simulink model "step6_3_setup_PID_test"  (R2021b)
settings: Solver=ode45  StartTime=0.0  StopTime=15  RelTol=1e-3  EnableMultiTasking=on
values from neighbouring files (symbols this model uses):
  adingain = [adin_gain 1 1 1 1 1]    [hwinit.m]    (also in hwinit_raw.m)
  adinoffs = [adin_offs 0 0 0 0 0]    [hwinit.m]    (also in hwinit_raw.m)
  daoutgain = 1*[-6]    [hwinit.m]    (also in hwinit_raw.m)
  daoutoffs = [0.00]    [hwinit.m]    (also in hwinit_raw.m)
  h = 0.001    [hwinit.m]    (also in hwinit_raw.m; init_fugi.m = fugiboard('Open', 'Pendulum1'); one_run.m = fugiboard('Open', 'pendulum1'); one_single_run.m = fugiboard('Open', 'pendulum1'))
  theta_1_0 = pi    (= 3.14159265359)    [hwinit.m]    (also in hwinit_raw.m; step4_0_linearize_operating_point.m; step5_observor_design.m = x_op(1); step6_1_controller_feedback.m = x_op(1))
  theta_2_0 = 0    [hwinit.m]    (also in hwinit_raw.m; step4_0_linearize_operating_point.m; step5_observor_design.m = x_op(3); step6_1_controller_feedback.m = x_op(3))
libraries: slpidlib x4
settings Model: Creator=rbabuska  LastModifiedBy=97083
settings SolverCC: AlgebraicLoopSolver=TrustRegion
settings DataIOCC: LimitDataPoints=on  SaveFormat=Array  ReturnWorkspaceOutputs=off  SignalLoggingName=sigsOut
settings OptimizationCC: BooleanDataType=off  ExpressionDepthLimit=2147483647  InitFltsAndDblsToZero=on  LifeSpan=inf
settings DebuggingCC: SaveWithParameterizedLinksMsg=none  SignalResolutionControl=TryResolveAllWithWarning  MultiTaskDSMMsg=warning  MultiTaskCondExecSysMsg=none  AllowSymbolicDim=off  StateNameClashWarn=warning  SFUnexpectedBacktrackingDiag=warning  SFNoUnconditionalDefaultTransitionDiag=warning  SFExecutionAtInitializationDiag=none  SFMachineParentedDataDiag=warning  ArithmeticOperatorsInVariantConditions=warning
settings HardwareCC: ProdBitPerPointer=32  ProdBitPerSizeT=32  ProdBitPerPtrDiffT=32  ProdLargestAtomicFloat=None  ProdIntDivRoundTo=Undefined  ProdEndianess=Unspecified  ProdWordSize=32  ProdHWDeviceType=32-bit Generic  TargetUnknown=on
settings ModelReferenceCC: PropagateSignalLabelsOutOfModel=off
settings SFSimCC: SimUseLocalCustomCode=off  CustomCodeUndefinedFunction=UseInterfaceOnly
settings RTWCC: RTWUseLocalCustomCode=off
settings CodeAppCC: StateflowObjectComments=on
settings GRTTargetCC: TargetFcnLib=ansi_tfl_tmw.mat  TargetLangStandard=C89/C90 (ANSI)  CombineOutputUpdateFcns=off  GRTInterface=on
settings ConfigComp: CovMetricSettings=dw  CovSaveCumulativeToWorkspaceVar=on  CovSaveSingleToWorkspaceVar=on  CovExternalEMLEnable=off

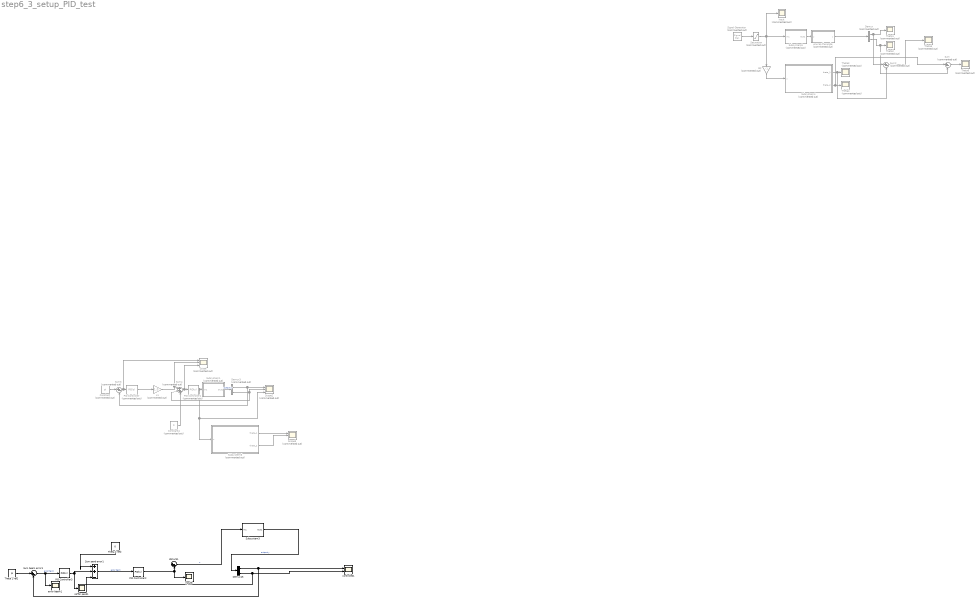
== system step6_3_setup_PID_test ==
  B2 : Gain  Commented=on  Gain=-1
  Constant : Constant  Commented=on  Value=pi
  Constant4 : Constant  Commented=on  Value=0
  Demux : Demux  Commented=on  Outputs=2
  Demux15 : Demux  Outputs=2
  Demux3 : Demux  Commented=on  Outputs=2
  Input : Scope  Commented=on
  L1 : Gain  Commented=on  Gain=1.0
  PID Controller : slpidlib/PID Controller  Commented=on  Controller=PID  Form=Parallel  TimeDomain=Continuous-time  UseExternalTs=off  SampleTime=-1  IntegratorMethod=Forward Euler  FilterMethod=Forward Euler  ControllerParametersSource=internal  P=0.5  I=-0.1  D=-0.079  N=0.05  UseFilter=on  TunerSelectOption=Transfer Function Based (PID Tuner App)  InitialConditionSource=internal  InitialConditionForIntegrator=0  InitialConditionForFilter=0  DifferentiatorICPrevScaledInput=0  ExternalReset=none  TrackingMode=off  Kt=1  LimitOutput=off  SatLimitsSource=internal  UpperSaturationLimit=inf  LowerSaturationLimit=-inf  LinearizeAsGain=on  AntiWindupMode=none  Kb=1  POutMin=[]  POutMax=[]  IOutMin=[]  IOutMax=[]  DOutMin=[]  DOutMax=[]  NOutMin=[]  NOutMax=[]  SumOutMin=[]  SumOutMax=[]  SaturationOutMin=[]  SaturationOutMax=[]  PParamMin=[]  PParamMax=[]  IParamMin=[]  IParamMax=[]  DParamMin=[]  DParamMax=[]  NParamMin=[]  NParamMax=[]  KbParamMin=[]  KbParamMax=[]  KtParamMin=[]  KtParamMax=[]  KbOutMin=[]  KbOutMax=[]  KtOutMin=[]  KtOutMax=[]  IntegratorOutMin=[]  IntegratorOutMax=[]  FilterOutMin=[]  FilterOutMax=[]  SumI1OutMin=[]  SumI1OutMax=[]  SumI2OutMin=[]  SumI2OutMax=[]  SumI3OutMin=[]  SumI3OutMax=[]  SumI4OutMin=[]  SumI4OutMax=[]  SumDOutMin=[]  SumDOutMax=[]  DifferentiatorOutMin=[]  DifferentiatorOutMax=[]  FilterDiffOutCoefMin=[]  FilterDiffOutCoefMax=[]  ReciprocalOutMin=[]  ReciprocalOutMax=[]  SumDenOutMin=[]  SumDenOutMax=[]  SumNumOutMin=[]  SumNumOutMax=[]  DivideOutMin=[]  DivideOutMax=[]  UdiffTsProdOutMin=[]  UdiffTsProdOutMax=[]  NTsProdOutMin=[]  NTsProdOutMax=[]  UintegralTsProdOutMin=[]  UintegralTsProdOutMax=[]  UngainTsProdOutMin=[]  UngainTsProdOutMax=[]  IntegratorContinuousStateAttributes=''  IntegratorStateMustResolveToSignalObject=off  IntegratorRTWStateStorageClass=Auto  FilterContinuousStateAttributes=''  FilterStateMustResolveToSignalObject=off  FilterRTWStateStorageClass=Auto  ParallelPVariant=InternalParameters  IdealPVariant=Disabled  IVariant=InternalParameters  DVariant=InternalParameters  IntegratorVariant=Continuous  SatVariant=Disabled  AWVariant=Passthrough  PCopyVariant=Disabled  TRVariant=Disabled  FdbkBlocksVariant=Forward  IdealPFdbkVariant=Disabled  SatFdbkVariant=Disabled  DerivativeFilterVariant=ContFilter  NVariant=InternalParameters  NCopyVariant=Disabled  FilterICVariant=InternalICsFilter  IntegratorICVariant=InternalICs  ExternalResetVariant=Disabled  TRSumVariant=Passthrough  SumFdbkVariant=Disabled  SumVariant=Sum_PID  TsampFilterVariant=InternalTs  TsampNgainVariant=Passthrough  TsampIntegralVariant=Passthrough  ExternalSaturationOutDataTypeStr=Inherit: Same as second input
  PID Controller1 : slpidlib/PID Controller  Commented=on  Controller=PID  Form=Parallel  TimeDomain=Continuous-time  UseExternalTs=off  SampleTime=-1  IntegratorMethod=Forward Euler  FilterMethod=Forward Euler  ControllerParametersSource=internal  P=3  I=0.1  D=0.0083  N=3  UseFilter=on  TunerSelectOption=Transfer Function Based (PID Tuner App)  InitialConditionSource=internal  InitialConditionForIntegrator=0  InitialConditionForFilter=0  DifferentiatorICPrevScaledInput=0  ExternalReset=none  TrackingMode=off  Kt=1  LimitOutput=off  SatLimitsSource=internal  UpperSaturationLimit=inf  LowerSaturationLimit=-inf  LinearizeAsGain=on  AntiWindupMode=none  Kb=1  POutMin=[]  POutMax=[]  IOutMin=[]  IOutMax=[]  DOutMin=[]  DOutMax=[]  NOutMin=[]  NOutMax=[]  SumOutMin=[]  SumOutMax=[]  SaturationOutMin=[]  SaturationOutMax=[]  PParamMin=[]  PParamMax=[]  IParamMin=[]  IParamMax=[]  DParamMin=[]  DParamMax=[]  NParamMin=[]  NParamMax=[]  KbParamMin=[]  KbParamMax=[]  KtParamMin=[]  KtParamMax=[]  KbOutMin=[]  KbOutMax=[]  KtOutMin=[]  KtOutMax=[]  IntegratorOutMin=[]  IntegratorOutMax=[]  FilterOutMin=[]  FilterOutMax=[]  SumI1OutMin=[]  SumI1OutMax=[]  SumI2OutMin=[]  SumI2OutMax=[]  SumI3OutMin=[]  SumI3OutMax=[]  SumI4OutMin=[]  SumI4OutMax=[]  SumDOutMin=[]  SumDOutMax=[]  DifferentiatorOutMin=[]  DifferentiatorOutMax=[]  FilterDiffOutCoefMin=[]  FilterDiffOutCoefMax=[]  ReciprocalOutMin=[]  ReciprocalOutMax=[]  SumDenOutMin=[]  SumDenOutMax=[]  SumNumOutMin=[]  SumNumOutMax=[]  DivideOutMin=[]  DivideOutMax=[]  UdiffTsProdOutMin=[]  UdiffTsProdOutMax=[]  NTsProdOutMin=[]  NTsProdOutMax=[]  UintegralTsProdOutMin=[]  UintegralTsProdOutMax=[]  UngainTsProdOutMin=[]  UngainTsProdOutMax=[]  IntegratorContinuousStateAttributes=''  IntegratorStateMustResolveToSignalObject=off  IntegratorRTWStateStorageClass=Auto  FilterContinuousStateAttributes=''  FilterStateMustResolveToSignalObject=off  FilterRTWStateStorageClass=Auto  ParallelPVariant=InternalParameters  IdealPVariant=Disabled  IVariant=InternalParameters  DVariant=InternalParameters  IntegratorVariant=Continuous  SatVariant=Disabled  AWVariant=Passthrough  PCopyVariant=Disabled  TRVariant=Disabled  FdbkBlocksVariant=Forward  IdealPFdbkVariant=Disabled  SatFdbkVariant=Disabled  DerivativeFilterVariant=ContFilter  NVariant=InternalParameters  NCopyVariant=Disabled  FilterICVariant=InternalICsFilter  IntegratorICVariant=InternalICs  ExternalResetVariant=Disabled  TRSumVariant=Passthrough  SumFdbkVariant=Disabled  SumVariant=Sum_PID  TsampFilterVariant=InternalTs  TsampNgainVariant=Passthrough  TsampIntegralVariant=Passthrough  ExternalSaturationOutDataTypeStr=Inherit: Same as second input
  PID Controller2 : slpidlib/PID Controller  Controller=PID  Form=Parallel  TimeDomain=Continuous-time  UseExternalTs=off  SampleTime=-1  IntegratorMethod=Forward Euler  FilterMethod=Forward Euler  ControllerParametersSource=internal  P=3  I=0.1  D=0.0083  N=3  UseFilter=on  TunerSelectOption=Transfer Function Based (PID Tuner App)  InitialConditionSource=internal  InitialConditionForIntegrator=0  InitialConditionForFilter=0  DifferentiatorICPrevScaledInput=0  ExternalReset=none  TrackingMode=off  Kt=1  LimitOutput=off  SatLimitsSource=internal  UpperSaturationLimit=inf  LowerSaturationLimit=-inf  LinearizeAsGain=on  AntiWindupMode=none  Kb=1  POutMin=[]  POutMax=[]  IOutMin=[]  IOutMax=[]  DOutMin=[]  DOutMax=[]  NOutMin=[]  NOutMax=[]  SumOutMin=[]  SumOutMax=[]  SaturationOutMin=[]  SaturationOutMax=[]  PParamMin=[]  PParamMax=[]  IParamMin=[]  IParamMax=[]  DParamMin=[]  DParamMax=[]  NParamMin=[]  NParamMax=[]  KbParamMin=[]  KbParamMax=[]  KtParamMin=[]  KtParamMax=[]  KbOutMin=[]  KbOutMax=[]  KtOutMin=[]  KtOutMax=[]  IntegratorOutMin=[]  IntegratorOutMax=[]  FilterOutMin=[]  FilterOutMax=[]  SumI1OutMin=[]  SumI1OutMax=[]  SumI2OutMin=[]  SumI2OutMax=[]  SumI3OutMin=[]  SumI3OutMax=[]  SumI4OutMin=[]  SumI4OutMax=[]  SumDOutMin=[]  SumDOutMax=[]  DifferentiatorOutMin=[]  DifferentiatorOutMax=[]  FilterDiffOutCoefMin=[]  FilterDiffOutCoefMax=[]  ReciprocalOutMin=[]  ReciprocalOutMax=[]  SumDenOutMin=[]  SumDenOutMax=[]  SumNumOutMin=[]  SumNumOutMax=[]  DivideOutMin=[]  DivideOutMax=[]  UdiffTsProdOutMin=[]  UdiffTsProdOutMax=[]  NTsProdOutMin=[]  NTsProdOutMax=[]  UintegralTsProdOutMin=[]  UintegralTsProdOutMax=[]  UngainTsProdOutMin=[]  UngainTsProdOutMax=[]  IntegratorContinuousStateAttributes=''  IntegratorStateMustResolveToSignalObject=off  IntegratorRTWStateStorageClass=Auto  FilterContinuousStateAttributes=''  FilterStateMustResolveToSignalObject=off  FilterRTWStateStorageClass=Auto  ParallelPVariant=InternalParameters  IdealPVariant=Disabled  IVariant=InternalParameters  DVariant=InternalParameters  IntegratorVariant=Continuous  SatVariant=Disabled  AWVariant=Passthrough  PCopyVariant=Disabled  TRVariant=Disabled  FdbkBlocksVariant=Forward  IdealPFdbkVariant=Disabled  SatFdbkVariant=Disabled  DerivativeFilterVariant=ContFilter  NVariant=InternalParameters  NCopyVariant=Disabled  FilterICVariant=InternalICsFilter  IntegratorICVariant=InternalICs  ExternalResetVariant=Disabled  TRSumVariant=Passthrough  SumFdbkVariant=Disabled  SumVariant=Sum_PID  TsampFilterVariant=InternalTs  TsampNgainVariant=Passthrough  TsampIntegralVariant=Passthrough  ExternalSaturationOutDataTypeStr=Inherit: Same as second input
  PID Controller3 : slpidlib/PID Controller  Controller=PID  Form=Parallel  TimeDomain=Continuous-time  UseExternalTs=off  SampleTime=-1  IntegratorMethod=Forward Euler  FilterMethod=Forward Euler  ControllerParametersSource=internal  P=0.5  I=-0.1  D=-0.079  N=0.05  UseFilter=on  TunerSelectOption=Transfer Function Based (PID Tuner App)  InitialConditionSource=internal  InitialConditionForIntegrator=0  InitialConditionForFilter=0  DifferentiatorICPrevScaledInput=0  ExternalReset=none  TrackingMode=off  Kt=1  LimitOutput=off  SatLimitsSource=internal  UpperSaturationLimit=inf  LowerSaturationLimit=-inf  LinearizeAsGain=on  AntiWindupMode=none  Kb=1  POutMin=[]  POutMax=[]  IOutMin=[]  IOutMax=[]  DOutMin=[]  DOutMax=[]  NOutMin=[]  NOutMax=[]  SumOutMin=[]  SumOutMax=[]  SaturationOutMin=[]  SaturationOutMax=[]  PParamMin=[]  PParamMax=[]  IParamMin=[]  IParamMax=[]  DParamMin=[]  DParamMax=[]  NParamMin=[]  NParamMax=[]  KbParamMin=[]  KbParamMax=[]  KtParamMin=[]  KtParamMax=[]  KbOutMin=[]  KbOutMax=[]  KtOutMin=[]  KtOutMax=[]  IntegratorOutMin=[]  IntegratorOutMax=[]  FilterOutMin=[]  FilterOutMax=[]  SumI1OutMin=[]  SumI1OutMax=[]  SumI2OutMin=[]  SumI2OutMax=[]  SumI3OutMin=[]  SumI3OutMax=[]  SumI4OutMin=[]  SumI4OutMax=[]  SumDOutMin=[]  SumDOutMax=[]  DifferentiatorOutMin=[]  DifferentiatorOutMax=[]  FilterDiffOutCoefMin=[]  FilterDiffOutCoefMax=[]  ReciprocalOutMin=[]  ReciprocalOutMax=[]  SumDenOutMin=[]  SumDenOutMax=[]  SumNumOutMin=[]  SumNumOutMax=[]  DivideOutMin=[]  DivideOutMax=[]  UdiffTsProdOutMin=[]  UdiffTsProdOutMax=[]  NTsProdOutMin=[]  NTsProdOutMax=[]  UintegralTsProdOutMin=[]  UintegralTsProdOutMax=[]  UngainTsProdOutMin=[]  UngainTsProdOutMax=[]  IntegratorContinuousStateAttributes=''  IntegratorStateMustResolveToSignalObject=off  IntegratorRTWStateStorageClass=Auto  FilterContinuousStateAttributes=''  FilterStateMustResolveToSignalObject=off  FilterRTWStateStorageClass=Auto  ParallelPVariant=InternalParameters  IdealPVariant=Disabled  IVariant=InternalParameters  DVariant=InternalParameters  IntegratorVariant=Continuous  SatVariant=Disabled  AWVariant=Passthrough  PCopyVariant=Disabled  TRVariant=Disabled  FdbkBlocksVariant=Forward  IdealPFdbkVariant=Disabled  SatFdbkVariant=Disabled  DerivativeFilterVariant=ContFilter  NVariant=InternalParameters  NCopyVariant=Disabled  FilterICVariant=InternalICsFilter  IntegratorICVariant=InternalICs  ExternalResetVariant=Disabled  TRSumVariant=Passthrough  SumFdbkVariant=Disabled  SumVariant=Sum_PID  TsampFilterVariant=InternalTs  TsampNgainVariant=Passthrough  TsampIntegralVariant=Passthrough  ExternalSaturationOutDataTypeStr=Inherit: Same as second input
  Saturation : Saturate  Commented=on  UpperLimit=1  LowerLimit=-1
  Scope : Scope  Commented=on  NumInputPorts=3
  Scope2 : Scope  Commented=on  NumInputPorts=3
  Scope3 : Scope  Commented=on  NumInputPorts=3
  Signal Generator : SignalGenerator  Commented=on  Amplitude=0.5  Frequency=[1]
  Subsystem1 : Subsystem  Commented=on
      mask Display: disp('Rotational\nPendulum')
  Subsystem3 : Subsystem
      mask Display: disp('Rotational\nPendulum')
  Subsystem4 : Subsystem  Commented=on
  Subsystem5 : Subsystem  Commented=on
      mask Display: disp('Rotational\nPendulum')
  Subsystem6 : Subsystem  Commented=on
  Sum : Sum  Commented=on  Inputs=|+-
  Sum beam error1 : Sum  Inputs=|+-
  Sum pend error1 : Sum  Inputs=|++-
  Sum2 : Sum  Commented=on  Inputs=|+-
  Sum3 : Sum  Commented=on  Inputs=|+-
  Sum4 : Sum  Commented=on  Inputs=|+-+
  Theta 1 ref2 : Constant  Value=pi
  Theta 2 ref2 : Constant  Value=0
  Theta{1..6} (6 alike) : Scope  Commented=on
  controled1 : Scope  NumInputPorts=2
  disturb1 : Sum  Inputs=|++
  error beam1 : Scope
  input8 : Scope
  ref for pend1 : Scope
  unwrap the angle : MATLAB Function  Commented=on  TreatAsAtomicUnit=on
  wires:
  Demux15/1 -> controled1/1, Sum beam error1/2
  Sum beam error1/1 -> PID Controller3/1, error beam1/1  "error term"
  disturb1/1 -> Subsystem3/1(In1)  "u"
  Theta 2 ref2/1 -> Sum pend error1/1
  Theta 1 ref2/1 -> Sum beam error1/1
  Demux15/2 -> Sum pend error1/3, controled1/2
  Sum pend error1/1 -> PID Controller2/1  "error term"
  PID Controller3/1 -> ref for pend1/1, Sum pend error1/2
  PID Controller2/1 -> input8/1, disturb1/2
  Subsystem3/1(Out1) -> Demux15/1  "output y"
  Demux/1 -> Theta1/1, Sum2/1
  Subsystem5/1(Out1) -> unwrap the angle/1(u)
  Signal Generator/1 -> Saturation/1
  Saturation/1 -> B2/1, Subsystem5/1(In1), Input/1
  Subsystem4/1(theta_1) -> Sum2/2, Theta3/1
  Subsystem4/2(theta_2) -> Sum/1, Theta4/1
  B2/1 -> Subsystem4/1(u)
  unwrap the angle/1(y) -> Demux/1
  Demux/2 -> Sum/2, Theta2/1
  Sum2/1 -> Theta5/1
  Sum/1 -> Theta6/1
  Subsystem1/1(Out1) -> Demux3/1  "output y"
  Sum4/1 -> Scope/3, PID Controller1/1
  PID Controller1/1 -> Scope2/3, Subsystem6/1(u), Subsystem1/1(In1)
  Sum3/1 -> Scope/1, PID Controller/1
  Constant/1 -> Sum3/1
  Demux3/2 -> Sum4/2, Scope2/2
  PID Controller/1 -> L1/1
  L1/1 -> Scope/2, Sum4/1
  Demux3/1 -> Scope2/1, Sum3/2
  Constant4/1 -> Sum4/3
  Subsystem6/1(theta_1) -> Scope3/1
  Subsystem6/2(theta_2) -> Scope3/2

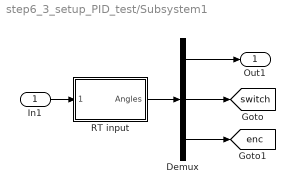
== system step6_3_setup_PID_test/Subsystem1 ==
  In1 : Inport
  Demux : Demux  Outputs=[2 4 1]
  RT input : Subsystem  mask{Ts=h, channels=[6 7]}
      mask prompts: Ts "Sample time [s]:"; channels "Channels to read (e.g., [6 7])"
      mask init:
      | hwinit;
      | 
      | % initialize FPGA
      | fugihandle = fugiboard('Open', 'Pendulum1');
      | fugihandle.WatchdogTimeout = 0.5;
      | fugiboard('SetParams', fugihandle);
      | fugiboard('Write', fugihandle, 0, 0, 0, 0);  % dummy write to sync interface board
      | fugiboard('Write', fugihandle, 5, 1, 0, 0);  % reset position, activate relay
      | data = fugiboard('Read', fugihandle);        % get version info from FPGA
      | % model = bitshift(data(1), -5); 
      | % version = bitand(data(1), 31);
      | % disp(sprintf('FPGA setup %d, version %d', model, version)); % for the B&P it should say 1 1, or else there is a problem
      | fugiboard('Write', fugihandle, 0, 1, 0, 0);  % end reset
      | pause(0.1);                         % give relay some time to respond
      mask Display: disp('Rotational\nPendulum')
  Out1 : Outport
  tag scope: enc=global, switch=global
  wires:
  RT input/1(Angles) -> Demux/1
  Demux/1 -> Out1/1
  Demux/2 -> [switch]
  Demux/3 -> [enc]
  In1/1 -> RT input/1(Motors)

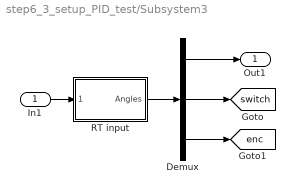
== system step6_3_setup_PID_test/Subsystem3 ==
  In1 : Inport
  Demux : Demux  Outputs=[2 4 1]
  RT input : Subsystem  mask{Ts=h, channels=[6 7]}
      mask prompts: Ts "Sample time [s]:"; channels "Channels to read (e.g., [6 7])"
      mask init: same as step6_3_setup_PID_test/Subsystem1/RT input
      mask Display: disp('Rotational\nPendulum')
  Out1 : Outport
  tag scope: enc=global, switch=global
  wires:
  RT input/1(Angles) -> Demux/1
  Demux/1 -> Out1/1
  Demux/2 -> [switch]
  Demux/3 -> [enc]
  In1/1 -> RT input/1(Motors)

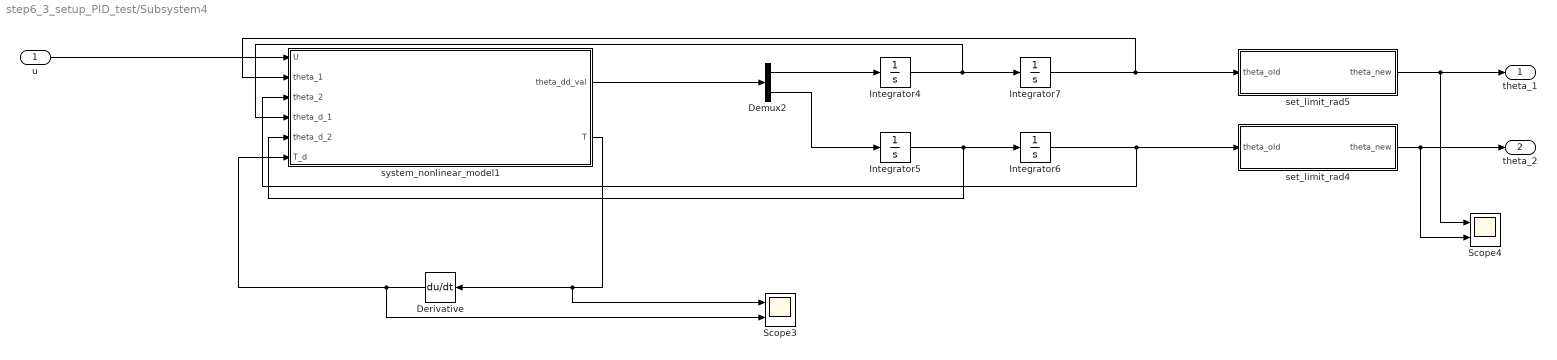
== system step6_3_setup_PID_test/Subsystem4 ==
  u : Inport
  Demux2 : Demux  Outputs=2
  Derivative : Derivative  CoefficientInTFapproximation=0
  Integrator4 : Integrator
  Integrator5 : Integrator
  Integrator6 : Integrator  InitialCondition=theta_2_0
  Integrator7 : Integrator  InitialCondition=theta_1_0
  Scope3 : Scope  NumInputPorts=2
  Scope4 : Scope  NumInputPorts=2
  set_limit_rad4 : MATLAB Function  TreatAsAtomicUnit=on
  set_limit_rad5 : MATLAB Function  TreatAsAtomicUnit=on
  system_nonlinear_model1 : MATLAB Function  TreatAsAtomicUnit=on
  theta_1 : Outport
  theta_2 : Outport  Port=2
  wires:
  Derivative/1 -> Scope3/2, system_nonlinear_model1/6(T_d)
  system_nonlinear_model1/2(T) -> Scope3/1, Derivative/1
  set_limit_rad4/1(theta_new) -> theta_2/1, Scope4/2
  Integrator4/1 -> system_nonlinear_model1/4(theta_d_1), Integrator7/1
  system_nonlinear_model1/1(theta_dd_val) -> Demux2/1
  Integrator6/1 -> system_nonlinear_model1/3(theta_2), set_limit_rad4/1(theta_old)
  u/1 -> system_nonlinear_model1/1(U)
  Integrator7/1 -> set_limit_rad5/1(theta_old), system_nonlinear_model1/2(theta_1)
  Integrator5/1 -> system_nonlinear_model1/5(theta_d_2), Integrator6/1
  Demux2/1 -> Integrator4/1
  Demux2/2 -> Integrator5/1
  set_limit_rad5/1(theta_new) -> theta_1/1, Scope4/1

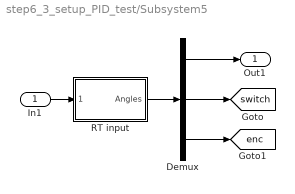
== system step6_3_setup_PID_test/Subsystem5 ==
  In1 : Inport
  Demux : Demux  Outputs=[2 4 1]
  RT input : Subsystem  mask{Ts=h, channels=[6 7]}
      mask prompts: Ts "Sample time [s]:"; channels "Channels to read (e.g., [6 7])"
      mask init: same as step6_3_setup_PID_test/Subsystem1/RT input
      mask Display: disp('Rotational\nPendulum')
  Out1 : Outport
  tag scope: enc=global, switch=global
  wires:
  RT input/1(Angles) -> Demux/1
  Demux/1 -> Out1/1
  Demux/2 -> [switch]
  Demux/3 -> [enc]
  In1/1 -> RT input/1(Motors)

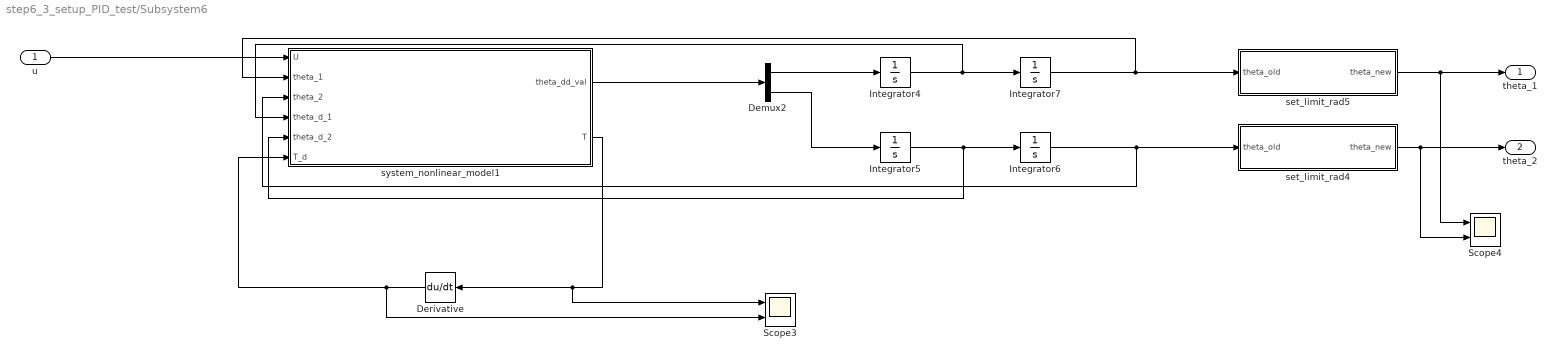
== system step6_3_setup_PID_test/Subsystem6 ==
  u : Inport
  Demux2 : Demux  Outputs=2
  Derivative : Derivative  CoefficientInTFapproximation=0
  Integrator4 : Integrator
  Integrator5 : Integrator
  Integrator6 : Integrator  InitialCondition=theta_2_0
  Integrator7 : Integrator  InitialCondition=theta_1_0
  Scope3 : Scope  NumInputPorts=2
  Scope4 : Scope  NumInputPorts=2
  set_limit_rad4 : MATLAB Function  TreatAsAtomicUnit=on
  set_limit_rad5 : MATLAB Function  TreatAsAtomicUnit=on
  system_nonlinear_model1 : MATLAB Function  TreatAsAtomicUnit=on
  theta_1 : Outport
  theta_2 : Outport  Port=2
  wires:
  Derivative/1 -> Scope3/2, system_nonlinear_model1/6(T_d)
  system_nonlinear_model1/2(T) -> Scope3/1, Derivative/1
  set_limit_rad4/1(theta_new) -> theta_2/1, Scope4/2
  Integrator4/1 -> system_nonlinear_model1/4(theta_d_1), Integrator7/1
  system_nonlinear_model1/1(theta_dd_val) -> Demux2/1
  Integrator6/1 -> system_nonlinear_model1/3(theta_2), set_limit_rad4/1(theta_old)
  u/1 -> system_nonlinear_model1/1(U)
  Integrator7/1 -> set_limit_rad5/1(theta_old), system_nonlinear_model1/2(theta_1)
  Integrator5/1 -> system_nonlinear_model1/5(theta_d_2), Integrator6/1
  Demux2/1 -> Integrator4/1
  Demux2/2 -> Integrator5/1
  set_limit_rad5/1(theta_new) -> theta_1/1, Scope4/1

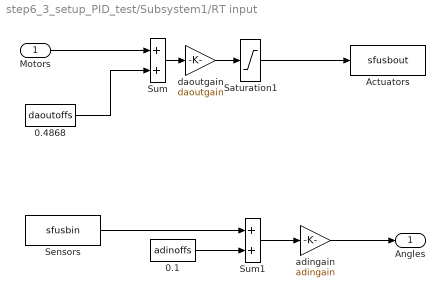
== system step6_3_setup_PID_test/Subsystem1/RT input ==
  Motors : Inport
  0.1 : Constant  Value=adinoffs
  0.4868 : Constant  Value=daoutoffs
  Actuators : S-Function  FunctionName=sfusbout  Parameters=Ts, fugihandle  SFunctionDeploymentMode=off  EnableBusSupport=off
  Saturation1 : Saturate  UpperLimit=10  LowerLimit=-10
  Sensors : S-Function  FunctionName=sfusbin  Parameters=Ts, fugihandle, channels  SFunctionDeploymentMode=off  EnableBusSupport=off
  Sum : Sum  InputSameDT=on  SaturateOnIntegerOverflow=on  OutDataTypeStr=Inherit: Same as first input
  Sum1 : Sum  InputSameDT=on  SaturateOnIntegerOverflow=on  OutDataTypeStr=Inherit: Same as first input
  adingain : Gain  Gain=adingain  SaturateOnIntegerOverflow=on  OutDataTypeStr=Inherit: Same as input  ParamDataTypeStr=Inherit: Same as input
  daoutgain : Gain  Gain=daoutgain  SaturateOnIntegerOverflow=on  OutDataTypeStr=Inherit: Same as input  ParamDataTypeStr=Inherit: Same as input
  Angles : Outport
  wires:
  Sum/1 -> daoutgain/1
  0.4868/1 -> Sum/2
  Motors/1 -> Sum/1
  Sum1/1 -> adingain/1
  0.1/1 -> Sum1/2
  adingain/1 -> Angles/1
  Saturation1/1 -> Actuators/1
  daoutgain/1 -> Saturation1/1
  Sensors/1 -> Sum1/1

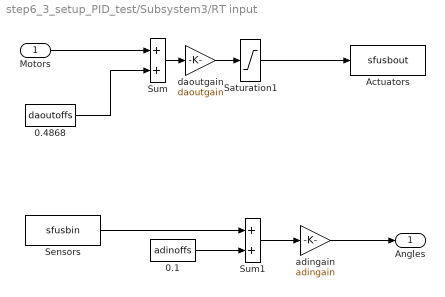
== system step6_3_setup_PID_test/Subsystem3/RT input ==
  Motors : Inport
  0.1 : Constant  Value=adinoffs
  0.4868 : Constant  Value=daoutoffs
  Actuators : S-Function  FunctionName=sfusbout  Parameters=Ts, fugihandle  SFunctionDeploymentMode=off  EnableBusSupport=off
  Saturation1 : Saturate  UpperLimit=10  LowerLimit=-10
  Sensors : S-Function  FunctionName=sfusbin  Parameters=Ts, fugihandle, channels  SFunctionDeploymentMode=off  EnableBusSupport=off
  Sum : Sum  InputSameDT=on  SaturateOnIntegerOverflow=on  OutDataTypeStr=Inherit: Same as first input
  Sum1 : Sum  InputSameDT=on  SaturateOnIntegerOverflow=on  OutDataTypeStr=Inherit: Same as first input
  adingain : Gain  Gain=adingain  SaturateOnIntegerOverflow=on  OutDataTypeStr=Inherit: Same as input  ParamDataTypeStr=Inherit: Same as input
  daoutgain : Gain  Gain=daoutgain  SaturateOnIntegerOverflow=on  OutDataTypeStr=Inherit: Same as input  ParamDataTypeStr=Inherit: Same as input
  Angles : Outport
  wires:
  Sum/1 -> daoutgain/1
  0.4868/1 -> Sum/2
  Motors/1 -> Sum/1
  Sum1/1 -> adingain/1
  0.1/1 -> Sum1/2
  adingain/1 -> Angles/1
  Saturation1/1 -> Actuators/1
  daoutgain/1 -> Saturation1/1
  Sensors/1 -> Sum1/1

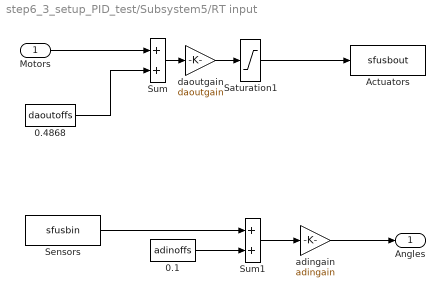
== system step6_3_setup_PID_test/Subsystem5/RT input ==
  Motors : Inport
  0.1 : Constant  Value=adinoffs
  0.4868 : Constant  Value=daoutoffs
  Actuators : S-Function  FunctionName=sfusbout  Parameters=Ts, fugihandle  SFunctionDeploymentMode=off  EnableBusSupport=off
  Saturation1 : Saturate  UpperLimit=10  LowerLimit=-10
  Sensors : S-Function  FunctionName=sfusbin  Parameters=Ts, fugihandle, channels  SFunctionDeploymentMode=off  EnableBusSupport=off
  Sum : Sum  InputSameDT=on  SaturateOnIntegerOverflow=on  OutDataTypeStr=Inherit: Same as first input
  Sum1 : Sum  InputSameDT=on  SaturateOnIntegerOverflow=on  OutDataTypeStr=Inherit: Same as first input
  adingain : Gain  Gain=adingain  SaturateOnIntegerOverflow=on  OutDataTypeStr=Inherit: Same as input  ParamDataTypeStr=Inherit: Same as input
  daoutgain : Gain  Gain=daoutgain  SaturateOnIntegerOverflow=on  OutDataTypeStr=Inherit: Same as input  ParamDataTypeStr=Inherit: Same as input
  Angles : Outport
  wires:
  Sum/1 -> daoutgain/1
  0.4868/1 -> Sum/2
  Motors/1 -> Sum/1
  Sum1/1 -> adingain/1
  0.1/1 -> Sum1/2
  adingain/1 -> Angles/1
  Saturation1/1 -> Actuators/1
  daoutgain/1 -> Saturation1/1
  Sensors/1 -> Sum1/1

== matlab function step6_3_setup_PID_test/Subsystem6/set_limit_rad4 ==
  settings: updateMethod=DISCRETE  sampleTime=0.001
  data: theta_old input size=1; theta_new output size=1
function theta_new   = set_limit_rad(theta_old)

% theta_new = theta_old - floor(theta_old / 2 / pi) * 2 * pi;
theta_new = theta_old;

== matlab function step6_3_setup_PID_test/Subsystem6/set_limit_rad5 ==
  settings: updateMethod=DISCRETE  sampleTime=0.001
  data: theta_old input size=1; theta_new output size=1
function theta_new   = set_limit_rad(theta_old)

% theta_new = theta_old - floor(theta_old / 2 / pi) * 2 * pi;
theta_new = theta_old;

== matlab function step6_3_setup_PID_test/Subsystem6/system_nonlinear_model1 ==
  settings: updateMethod=DISCRETE  sampleTime=0.001
  data: U input size=1; theta_dd_val output size=2; T output; theta_1 input size=1; theta_2 input size=1; theta_d_1 input size=1; theta_d_2 input size=1; T_d input
function [theta_dd_val, T]   = get_theta_dt_dt(U, theta_1, theta_2, theta_d_1, theta_d_2, T_d)


u = U(1);
k_m_0 = 65.9998023466922;
tau_e_0 = 0.003;
T = k_m_0 * u - tau_e_0 * T_d;

params = [-0.0300000121036330, 0.0203451968350115, 0.1000000000017210, 2.00882387117299e-05, 10.27570530021582, 0.78577414601457e-05, 49.9998023466922, 0.01500000000002200];  %found via white-box
% params = [-0.0984, 0.076, 0.074, 0.000045, 28.07, 0.000045, 25.9, 0.03];  %found via white-box
c_1_0 = params(1);
c_2_0 = params(2);
I_1_0 = params(3);
I_2_0 = params(4);
b_1_0 = params(5);
b_2_0 = params(6);





theta_dd_val = [
                                                                                                                                                                                                               theta_d_2*((200*b_2_0*(10*c_2_0^2 + cos(theta_2)*c_2_0 + 200*I_2_0))/(20*I_2_0 - c_2_0^2*cos(theta_2)^2 + 2000*I_1_0*c_2_0^2 + 5000*I_2_0*c_1_0^2 + c_2_0^2 + 250*c_1_0^2*c_2_0^2 + 40000*I_1_0*I_2_0) + (10*c_2_0*sin(theta_2)*(theta_d_1 + theta_d_2)*(c_2_0^2 + 20*I_2_0))/(20*I_2_0 - c_2_0^2*cos(theta_2)^2 + 2000*I_1_0*c_2_0^2 + 5000*I_2_0*c_1_0^2 + c_2_0^2 + 250*c_1_0^2*c_2_0^2 + 40000*I_1_0*I_2_0)) - theta_d_1*((2000*(c_2_0^2 + 20*I_2_0)*(b_1_0 - (c_2_0*theta_d_2*sin(theta_2))/200))/(20*I_2_0 - c_2_0^2*cos(theta_2)^2 + 2000*I_1_0*c_2_0^2 + 5000*I_2_0*c_1_0^2 + c_2_0^2 + 250*c_1_0^2*c_2_0^2 + 40000*I_1_0*I_2_0) - (c_2_0*theta_d_1*sin(theta_2)*(10*c_2_0^2 + cos(theta_2)*c_2_0 + 200*I_2_0))/(20*I_2_0 - c_2_0^2*cos(theta_2)^2 + 2000*I_1_0*c_2_0^2 + 5000*I_2_0*c_1_0^2 + c_2_0^2 + 250*c_1_0^2*c_2_0^2 + 40000*I_1_0*I_2_0)) + (2000*(sin(theta_1)*((981*c_1_0)/800 + 981/20000) + (981*c_2_0*sin(theta_1 + theta_2))/2000)*(c_2_0^2 + 20*I_2_0))/(20*I_2_0 - c_2_0^2*cos(theta_2)^2 + 2000*I_1_0*c_2_0^2 + 5000*I_2_0*c_1_0^2 + c_2_0^2 + 250*c_1_0^2*c_2_0^2 + 40000*I_1_0*I_2_0) + (2000*T*(c_2_0^2 + 20*I_2_0))/(20*I_2_0 - c_2_0^2*cos(theta_2)^2 + 2000*I_1_0*c_2_0^2 + 5000*I_2_0*c_1_0^2 + c_2_0^2 + 250*c_1_0^2*c_2_0^2 + 40000*I_1_0*I_2_0) - (981*c_2_0*sin(theta_1 + theta_2)*(10*c_2_0^2 + cos(theta_2)*c_2_0 + 200*I_2_0))/(10*(20*I_2_0 - c_2_0^2*cos(theta_2)^2 + 2000*I_1_0*c_2_0^2 + 5000*I_2_0*c_1_0^2 + c_2_0^2 + 250*c_1_0^2*c_2_0^2 + 40000*I_1_0*I_2_0))
theta_d_1*((200*(b_1_0 - (c_2_0*theta_d_2*sin(theta_2))/200)*(10*c_2_0^2 + cos(theta_2)*c_2_0 + 200*I_2_0))/(20*I_2_0 - c_2_0^2*cos(theta_2)^2 + 2000*I_1_0*c_2_0^2 + 5000*I_2_0*c_1_0^2 + c_2_0^2 + 250*c_1_0^2*c_2_0^2 + 40000*I_1_0*I_2_0) - (c_2_0*theta_d_1*sin(theta_2)*(250*c_1_0^2 + 100*c_2_0^2 + 20*cos(theta_2)*c_2_0 + 2000*I_1_0 + 2000*I_2_0 + 1))/(10*(20*I_2_0 - c_2_0^2*cos(theta_2)^2 + 2000*I_1_0*c_2_0^2 + 5000*I_2_0*c_1_0^2 + c_2_0^2 + 250*c_1_0^2*c_2_0^2 + 40000*I_1_0*I_2_0))) - theta_d_2*((20*b_2_0*(250*c_1_0^2 + 100*c_2_0^2 + 20*cos(theta_2)*c_2_0 + 2000*I_1_0 + 2000*I_2_0 + 1))/(20*I_2_0 - c_2_0^2*cos(theta_2)^2 + 2000*I_1_0*c_2_0^2 + 5000*I_2_0*c_1_0^2 + c_2_0^2 + 250*c_1_0^2*c_2_0^2 + 40000*I_1_0*I_2_0) + (c_2_0*sin(theta_2)*(theta_d_1 + theta_d_2)*(10*c_2_0^2 + cos(theta_2)*c_2_0 + 200*I_2_0))/(20*I_2_0 - c_2_0^2*cos(theta_2)^2 + 2000*I_1_0*c_2_0^2 + 5000*I_2_0*c_1_0^2 + c_2_0^2 + 250*c_1_0^2*c_2_0^2 + 40000*I_1_0*I_2_0)) - (200*(sin(theta_1)*((981*c_1_0)/800 + 981/20000) + (981*c_2_0*sin(theta_1 + theta_2))/2000)*(10*c_2_0^2 + cos(theta_2)*c_2_0 + 200*I_2_0))/(20*I_2_0 - c_2_0^2*cos(theta_2)^2 + 2000*I_1_0*c_2_0^2 + 5000*I_2_0*c_1_0^2 + c_2_0^2 + 250*c_1_0^2*c_2_0^2 + 40000*I_1_0*I_2_0) - (200*T*(10*c_2_0^2 + cos(theta_2)*c_2_0 + 200*I_2_0))/(20*I_2_0 - c_2_0^2*cos(theta_2)^2 + 2000*I_1_0*c_2_0^2 + 5000*I_2_0*c_1_0^2 + c_2_0^2 + 250*c_1_0^2*c_2_0^2 + 40000*I_1_0*I_2_0) + (981*c_2_0*sin(theta_1 + theta_2)*(250*c_1_0^2 + 100*c_2_0^2 + 20*cos(theta_2)*c_2_0 + 2000*I_1_0 + 2000*I_2_0 + 1))/(100*(20*I_2_0 - c_2_0^2*cos(theta_2)^2 + 2000*I_1_0*c_2_0^2 + 5000*I_2_0*c_1_0^2 + c_2_0^2 + 250*c_1_0^2*c_2_0^2 + 40000*I_1_0*I_2_0));
];

== matlab function step6_3_setup_PID_test/Subsystem4/system_nonlinear_model1 ==
  settings: updateMethod=DISCRETE  sampleTime=0.001
  data: U input size=1; theta_dd_val output size=2; T output; theta_1 input size=1; theta_2 input size=1; theta_d_1 input size=1; theta_d_2 input size=1; T_d input
function [theta_dd_val, T]   = get_theta_dt_dt(U, theta_1, theta_2, theta_d_1, theta_d_2, T_d)


u = U(1);
k_m_0 = 65.9998023466922;
tau_e_0 = 0.003;
T = k_m_0 * u - tau_e_0 * T_d;

params = [-0.0300000121036330, 0.0203451968350115, 0.1000000000017210, 2.00882387117299e-05, 10.27570530021582, 0.78577414601457e-05, 49.9998023466922, 0.01500000000002200];  %found via white-box
% params = [-0.0984, 0.076, 0.074, 0.000045, 28.07, 0.000045, 25.9, 0.03];  %found via white-box
c_1_0 = params(1);
c_2_0 = params(2);
I_1_0 = params(3);
I_2_0 = params(4);
b_1_0 = params(5);
b_2_0 = params(6);





theta_dd_val = [
                                                                                                                                                                                                               theta_d_2*((200*b_2_0*(10*c_2_0^2 + cos(theta_2)*c_2_0 + 200*I_2_0))/(20*I_2_0 - c_2_0^2*cos(theta_2)^2 + 2000*I_1_0*c_2_0^2 + 5000*I_2_0*c_1_0^2 + c_2_0^2 + 250*c_1_0^2*c_2_0^2 + 40000*I_1_0*I_2_0) + (10*c_2_0*sin(theta_2)*(theta_d_1 + theta_d_2)*(c_2_0^2 + 20*I_2_0))/(20*I_2_0 - c_2_0^2*cos(theta_2)^2 + 2000*I_1_0*c_2_0^2 + 5000*I_2_0*c_1_0^2 + c_2_0^2 + 250*c_1_0^2*c_2_0^2 + 40000*I_1_0*I_2_0)) - theta_d_1*((2000*(c_2_0^2 + 20*I_2_0)*(b_1_0 - (c_2_0*theta_d_2*sin(theta_2))/200))/(20*I_2_0 - c_2_0^2*cos(theta_2)^2 + 2000*I_1_0*c_2_0^2 + 5000*I_2_0*c_1_0^2 + c_2_0^2 + 250*c_1_0^2*c_2_0^2 + 40000*I_1_0*I_2_0) - (c_2_0*theta_d_1*sin(theta_2)*(10*c_2_0^2 + cos(theta_2)*c_2_0 + 200*I_2_0))/(20*I_2_0 - c_2_0^2*cos(theta_2)^2 + 2000*I_1_0*c_2_0^2 + 5000*I_2_0*c_1_0^2 + c_2_0^2 + 250*c_1_0^2*c_2_0^2 + 40000*I_1_0*I_2_0)) + (2000*(sin(theta_1)*((981*c_1_0)/800 + 981/20000) + (981*c_2_0*sin(theta_1 + theta_2))/2000)*(c_2_0^2 + 20*I_2_0))/(20*I_2_0 - c_2_0^2*cos(theta_2)^2 + 2000*I_1_0*c_2_0^2 + 5000*I_2_0*c_1_0^2 + c_2_0^2 + 250*c_1_0^2*c_2_0^2 + 40000*I_1_0*I_2_0) + (2000*T*(c_2_0^2 + 20*I_2_0))/(20*I_2_0 - c_2_0^2*cos(theta_2)^2 + 2000*I_1_0*c_2_0^2 + 5000*I_2_0*c_1_0^2 + c_2_0^2 + 250*c_1_0^2*c_2_0^2 + 40000*I_1_0*I_2_0) - (981*c_2_0*sin(theta_1 + theta_2)*(10*c_2_0^2 + cos(theta_2)*c_2_0 + 200*I_2_0))/(10*(20*I_2_0 - c_2_0^2*cos(theta_2)^2 + 2000*I_1_0*c_2_0^2 + 5000*I_2_0*c_1_0^2 + c_2_0^2 + 250*c_1_0^2*c_2_0^2 + 40000*I_1_0*I_2_0))
theta_d_1*((200*(b_1_0 - (c_2_0*theta_d_2*sin(theta_2))/200)*(10*c_2_0^2 + cos(theta_2)*c_2_0 + 200*I_2_0))/(20*I_2_0 - c_2_0^2*cos(theta_2)^2 + 2000*I_1_0*c_2_0^2 + 5000*I_2_0*c_1_0^2 + c_2_0^2 + 250*c_1_0^2*c_2_0^2 + 40000*I_1_0*I_2_0) - (c_2_0*theta_d_1*sin(theta_2)*(250*c_1_0^2 + 100*c_2_0^2 + 20*cos(theta_2)*c_2_0 + 2000*I_1_0 + 2000*I_2_0 + 1))/(10*(20*I_2_0 - c_2_0^2*cos(theta_2)^2 + 2000*I_1_0*c_2_0^2 + 5000*I_2_0*c_1_0^2 + c_2_0^2 + 250*c_1_0^2*c_2_0^2 + 40000*I_1_0*I_2_0))) - theta_d_2*((20*b_2_0*(250*c_1_0^2 + 100*c_2_0^2 + 20*cos(theta_2)*c_2_0 + 2000*I_1_0 + 2000*I_2_0 + 1))/(20*I_2_0 - c_2_0^2*cos(theta_2)^2 + 2000*I_1_0*c_2_0^2 + 5000*I_2_0*c_1_0^2 + c_2_0^2 + 250*c_1_0^2*c_2_0^2 + 40000*I_1_0*I_2_0) + (c_2_0*sin(theta_2)*(theta_d_1 + theta_d_2)*(10*c_2_0^2 + cos(theta_2)*c_2_0 + 200*I_2_0))/(20*I_2_0 - c_2_0^2*cos(theta_2)^2 + 2000*I_1_0*c_2_0^2 + 5000*I_2_0*c_1_0^2 + c_2_0^2 + 250*c_1_0^2*c_2_0^2 + 40000*I_1_0*I_2_0)) - (200*(sin(theta_1)*((981*c_1_0)/800 + 981/20000) + (981*c_2_0*sin(theta_1 + theta_2))/2000)*(10*c_2_0^2 + cos(theta_2)*c_2_0 + 200*I_2_0))/(20*I_2_0 - c_2_0^2*cos(theta_2)^2 + 2000*I_1_0*c_2_0^2 + 5000*I_2_0*c_1_0^2 + c_2_0^2 + 250*c_1_0^2*c_2_0^2 + 40000*I_1_0*I_2_0) - (200*T*(10*c_2_0^2 + cos(theta_2)*c_2_0 + 200*I_2_0))/(20*I_2_0 - c_2_0^2*cos(theta_2)^2 + 2000*I_1_0*c_2_0^2 + 5000*I_2_0*c_1_0^2 + c_2_0^2 + 250*c_1_0^2*c_2_0^2 + 40000*I_1_0*I_2_0) + (981*c_2_0*sin(theta_1 + theta_2)*(250*c_1_0^2 + 100*c_2_0^2 + 20*cos(theta_2)*c_2_0 + 2000*I_1_0 + 2000*I_2_0 + 1))/(100*(20*I_2_0 - c_2_0^2*cos(theta_2)^2 + 2000*I_1_0*c_2_0^2 + 5000*I_2_0*c_1_0^2 + c_2_0^2 + 250*c_1_0^2*c_2_0^2 + 40000*I_1_0*I_2_0));
];

== matlab function step6_3_setup_PID_test/unwrap the angle ==
  settings: updateMethod=DISCRETE  sampleTime=0.001
  data: u input size=2; y output size=2
function y = unwrap_angle(u)

y = unwrap(u);
y = u;

== matlab function step6_3_setup_PID_test/Subsystem4/set_limit_rad4 ==
  settings: updateMethod=DISCRETE  sampleTime=0.001
  data: theta_old input size=1; theta_new output size=1
function theta_new   = set_limit_rad(theta_old)

% theta_new = theta_old - floor(theta_old / 2 / pi) * 2 * pi;
theta_new = theta_old;

== matlab function step6_3_setup_PID_test/Subsystem4/set_limit_rad5 ==
  settings: updateMethod=DISCRETE  sampleTime=0.001
  data: theta_old input size=1; theta_new output size=1
function theta_new   = set_limit_rad(theta_old)

% theta_new = theta_old - floor(theta_old / 2 / pi) * 2 * pi;
theta_new = theta_old;
